simulink model "slb_ram"  (R2015b)
settings: Solver=ode45  SolverMode=SingleTasking  StartTime=0.0  StopTime=1000  RelTol=1e-3
libraries: hdlsllib x4, dspsrcs4 x1, commutil2 x1
settings Model: Creator=amatsumo  LastModifiedBy=amatsumo
settings DataIOCC: SaveFormat=Array  SignalLogging=off
settings OptimizationCC: BlockReduction=off  ConditionallyExecuteInputs=off  DefaultParameterBehavior=Inlined
settings DebuggingCC: AlgebraicLoopMsg=error  SolverPrmCheckMsg=warning  SingleTaskRateTransMsg=error
settings HardwareCC: ProdBitPerPointer=32  ProdLargestAtomicFloat=None  ProdIntDivRoundTo=Undefined  ProdEndianess=Unspecified  ProdWordSize=32  ProdHWDeviceType=ASIC/FPGA->ASIC/FPGA  ProdEqTarget=off
settings GRTTargetCC: GeneratePreprocessorConditionals=Disable all
settings ConfigComp: CovModelRefEnable=Off  CovSFcnEnable=off

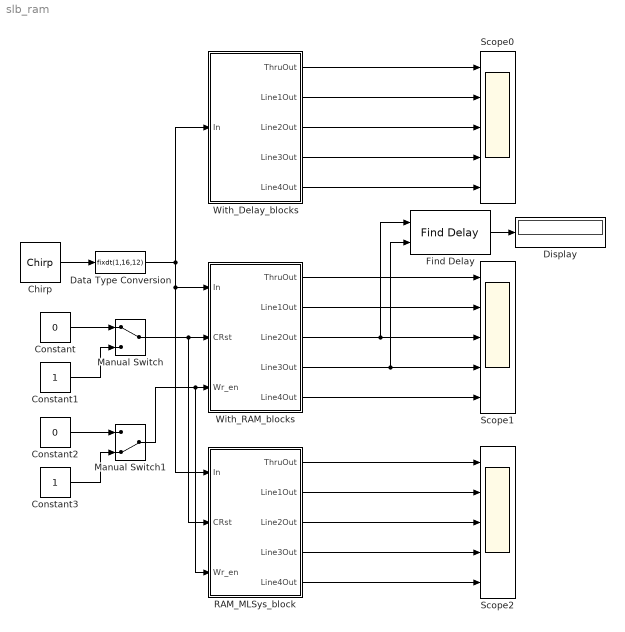
== system slb_ram ==
  Chirp : dspsrcs4/Chirp  sweep=Linear  mode=Unidirectional  f0=0.001  f1=0.1  t1=1000  Tsweep=1000  phase=0  Ts=1  spf=1  datatype=Double  OutputFrames=on
  Constant : Constant  Value=0  OutDataTypeStr=boolean  SampleTime=-1
  Constant1 : Constant  OutDataTypeStr=boolean  SampleTime=-1
  Constant2 : Constant  Value=0  OutDataTypeStr=boolean  SampleTime=-1
  Constant3 : Constant  OutDataTypeStr=boolean  SampleTime=-1
  Data Type Conversion : DataTypeConversion  OutDataTypeStr=fixdt(1,16,12)
  Display : Display
  Find Delay : commutil2/Find Delay  corrLength=600  chgSigOP=off  stopUpdate=off  numConstDelay=3
  Manual Switch : ManualSwitch
  Manual Switch1 : ManualSwitch  CurrentSetting=0
  RAM_MLSys_block : Subsystem
  Scope0 : Scope  NumInputPorts=5
  Scope1 : Scope  NumInputPorts=5
  Scope2 : Scope  NumInputPorts=5
  With_Delay_blocks : Subsystem
  With_RAM_blocks : Subsystem
  wires:
  Constant/1 -> Manual Switch/1
  Constant1/1 -> Manual Switch/2
  Manual Switch/1 -> RAM_MLSys_block/2(CRst), With_RAM_blocks/2(CRst)
  Chirp/1 -> Data Type Conversion/1
  With_RAM_blocks/1(ThruOut) -> Scope1/1
  With_RAM_blocks/2(Line1Out) -> Scope1/2
  With_RAM_blocks/3(Line2Out) -> Scope1/3, Find Delay/1
  With_RAM_blocks/4(Line3Out) -> Scope1/4, Find Delay/2
  With_RAM_blocks/5(Line4Out) -> Scope1/5
  Find Delay/1 -> Display/1
  Data Type Conversion/1 -> RAM_MLSys_block/1(In), With_RAM_blocks/1(In), With_Delay_blocks/1(In)
  Constant2/1 -> Manual Switch1/1
  Constant3/1 -> Manual Switch1/2
  Manual Switch1/1 -> RAM_MLSys_block/3(Wr_en), With_RAM_blocks/3(Wr_en)
  With_Delay_blocks/1(ThruOut) -> Scope0/1
  With_Delay_blocks/2(Line1Out) -> Scope0/2
  With_Delay_blocks/3(Line2Out) -> Scope0/3
  With_Delay_blocks/4(Line3Out) -> Scope0/4
  With_Delay_blocks/5(Line4Out) -> Scope0/5
  RAM_MLSys_block/1(ThruOut) -> Scope2/1
  RAM_MLSys_block/2(Line1Out) -> Scope2/2
  RAM_MLSys_block/3(Line2Out) -> Scope2/3
  RAM_MLSys_block/4(Line3Out) -> Scope2/4
  RAM_MLSys_block/5(Line4Out) -> Scope2/5

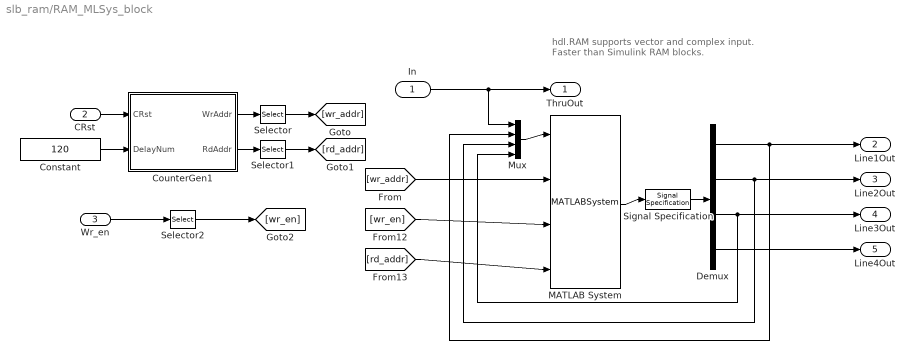
== system slb_ram/RAM_MLSys_block ==
  note: hdl.RAM supports vector and complex input.
      | Faster than Simulink RAM blocks.
  In : Inport
  CRst : Inport  Port=2
  Wr_en : Inport  Port=3
  Constant : Constant  Value=120  OutDataTypeStr=fixdt(0, ceil(log2(120+1)),0)  SampleTime=-1
  CounterGen1 : MATLAB Function  TreatAsAtomicUnit=on
  Demux : Demux
  MATLAB System : MATLABSystem  System=hdl.RAM  RAMType=Simple dual port  WriteOutputValue=New data  SimulateUsing=Code generation
      mask Type: hdl.RAM
      mask Display:
      | disp('RAM');
      | port_label('input',1,'din');
      | port_label('input',2,'wr_addr');
      | port_label('input',3,'wr_en');
      | port_label('input',4,'rd_addr');
      | port_label('output',1,'rd_dout');
  Mux : Mux
  Selector : Selector  InputPortWidth=1  IndexOptions=Index vector (dialog)  Indices=[1 1 1 1]  OutputSizes=1
  Selector1 : Selector  InputPortWidth=1  IndexOptions=Index vector (dialog)  Indices=[1 1 1 1]  OutputSizes=1
  Selector2 : Selector  InputPortWidth=1  IndexOptions=Index vector (dialog)  Indices=[1 1 1 1]  OutputSizes=1
  Signal Specification : SignalSpecification  Dimensions=[4 1]
  ThruOut : Outport
  Line1Out : Outport  Port=2
  Line2Out : Outport  Port=3
  Line3Out : Outport  Port=4
  Line4Out : Outport  Port=5
  wires:
  CounterGen1/2(RdAddr) -> Selector1/1
  CounterGen1/1(WrAddr) -> Selector/1
  Wr_en/1 -> Selector2/1
  Constant/1 -> CounterGen1/2(DelayNum)
  CRst/1 -> CounterGen1/1(CRst)
  Mux/1 -> MATLAB System/1
  MATLAB System/1 -> Signal Specification/1
  Demux/1 -> Line1Out/1, Mux/2
  In/1 -> Mux/1, ThruOut/1
  Demux/2 -> Line2Out/1, Mux/3
  Demux/3 -> Mux/4, Line3Out/1
  Demux/4 -> Line4Out/1
  [wr_addr] -> MATLAB System/2
  Selector/1 -> [wr_addr]
  Selector1/1 -> [rd_addr]
  Selector2/1 -> [wr_en]
  [rd_addr] -> MATLAB System/4
  [wr_en] -> MATLAB System/3
  Signal Specification/1 -> Demux/1

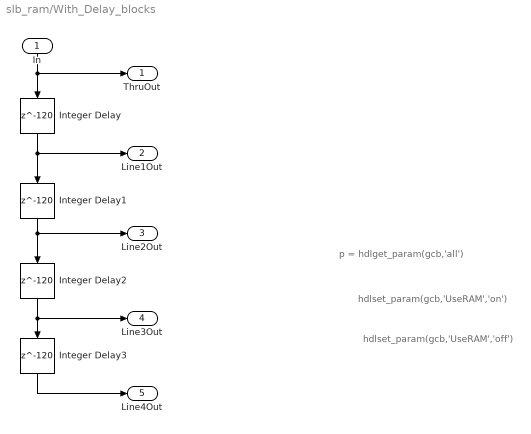
== system slb_ram/With_Delay_blocks ==
  note: hdlset_param(gcb,'UseRAM','off')
  note: hdlset_param(gcb,'UseRAM','on')
  note: p = hdlget_param(gcb,'all')
  In : Inport
  Integer Delay{,1..3} (4 alike) : Delay  DelayLength=120
  ThruOut : Outport
  Line1Out : Outport  Port=2
  Line2Out : Outport  Port=3
  Line3Out : Outport  Port=4
  Line4Out : Outport  Port=5
  wires:
  Integer Delay/1 -> Integer Delay1/1, Line1Out/1
  In/1 -> Integer Delay/1, ThruOut/1
  Integer Delay1/1 -> Integer Delay2/1, Line2Out/1
  Integer Delay2/1 -> Integer Delay3/1, Line3Out/1
  Integer Delay3/1 -> Line4Out/1

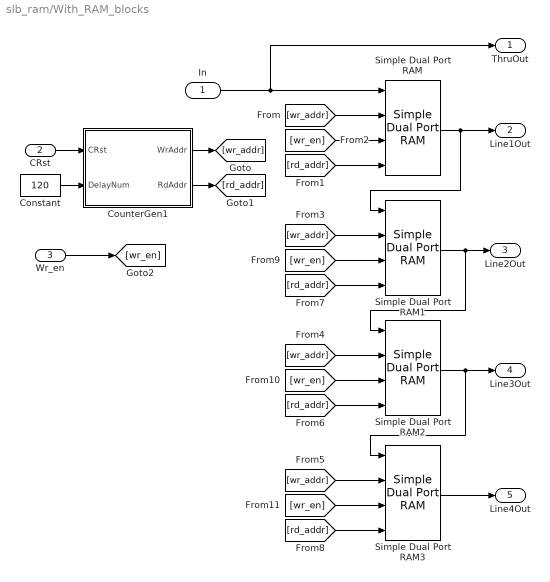
== system slb_ram/With_RAM_blocks ==
  In : Inport
  CRst : Inport  Port=2
  Wr_en : Inport  Port=3
  Constant : Constant  Value=120  OutDataTypeStr=uint8
  CounterGen1 : MATLAB Function  TreatAsAtomicUnit=on
  Simple Dual Port RAM{,1..3} (4 alike) : hdlsllib/HDL Operations/Simple Dual Port RAM  ram_size=8
  ThruOut : Outport
  Line1Out : Outport  Port=2
  Line2Out : Outport  Port=3
  Line3Out : Outport  Port=4
  Line4Out : Outport  Port=5
  wires:
  [wr_en] -> Simple Dual Port RAM3/3
  [wr_en] -> Simple Dual Port RAM2/3
  [wr_en] -> Simple Dual Port RAM1/3
  [wr_en] -> Simple Dual Port RAM/3
  [rd_addr] -> Simple Dual Port RAM3/4
  [rd_addr] -> Simple Dual Port RAM2/4
  [rd_addr] -> Simple Dual Port RAM1/4
  [rd_addr] -> Simple Dual Port RAM/4
  [wr_addr] -> Simple Dual Port RAM3/2
  [wr_addr] -> Simple Dual Port RAM2/2
  [wr_addr] -> Simple Dual Port RAM1/2
  [wr_addr] -> Simple Dual Port RAM/2
  CounterGen1/2(RdAddr) -> [rd_addr]
  CounterGen1/1(WrAddr) -> [wr_addr]
  Wr_en/1 -> [wr_en]
  Constant/1 -> CounterGen1/2(DelayNum)
  Simple Dual Port RAM3/1 -> Line4Out/1
  Simple Dual Port RAM2/1 -> Line3Out/1, Simple Dual Port RAM3/1
  Simple Dual Port RAM1/1 -> Line2Out/1, Simple Dual Port RAM2/1
  Simple Dual Port RAM/1 -> Line1Out/1, Simple Dual Port RAM1/1
  CRst/1 -> CounterGen1/1(CRst)
  In/1 -> ThruOut/1, Simple Dual Port RAM/1

== matlab function slb_ram/With_RAM_blocks/CounterGen1 ==
  data: WrAddr output; RdAddr output; CRst input boolean; DelayNum input
function [WrAddr,RdAddr] = counter(CRst, DelayNum)
% This block supports the Embedded MATLAB subset.
% See the help menu for details. 

% Parameters
% DelayNum=120;
UpperLim = DelayNum;

Type_nt = numerictype(0,8,0);
Type_fm = fimath('OverflowMode', 'wrap', 'RoundMode', 'floor');

persistent CountTemp

if isempty(CountTemp)
	CountTemp = fi(0,Type_nt, Type_fm);
end

% Output Count Down Signal
if ((CountTemp > 0)&&(CRst == 0))
	Temp = CountTemp-fi(1,Type_nt, Type_fm);
	CountTemp = fi(Temp, Type_nt, Type_fm);
else
	CountTemp = fi(UpperLim-1,Type_nt, Type_fm);
end

WrAddr = CountTemp;
if CountTemp <= 0
	Temp1 = fi(UpperLim-1,Type_nt, Type_fm);
	RdAddr = Temp1;
else
	Temp1 = fi(CountTemp-1,Type_nt, Type_fm);
	RdAddr = Temp1;
end

== matlab function slb_ram/RAM_MLSys_block/CounterGen1 ==
  data: WrAddr output; RdAddr output; CRst input boolean; DelayNum input
function [WrAddr,RdAddr] = counter(CRst, DelayNum)
% This block supports the Embedded MATLAB subset.
% See the help menu for details. 

% Parameters
% DelayNum=120;
UpperLim = DelayNum;

Type_nt = numerictype(0,8,0);
Type_fm = fimath('OverflowMode', 'wrap', 'RoundMode', 'floor');

persistent CountTemp

if isempty(CountTemp)
	CountTemp = fi(0,Type_nt, Type_fm);
end

% Output Count Down Signal
if ((CountTemp > 0)&&(CRst == 0))
	Temp = CountTemp-fi(1,Type_nt, Type_fm);
	CountTemp = fi(Temp, Type_nt, Type_fm);
else
	CountTemp = fi(UpperLim-1,Type_nt, Type_fm);
end

WrAddr = CountTemp;
if CountTemp <= 0
	Temp1 = fi(UpperLim-1,Type_nt, Type_fm);
	RdAddr = Temp1;
else
	Temp1 = fi(CountTemp-1,Type_nt, Type_fm);
	RdAddr = Temp1;
end
